simulink library "Lib_PF_LineEffAC_TMATS"  (R2017a)
settings: Solver=ode45  StartTime=0.0  StopTime=10.0  RelTol=1e-3  EnableMultiTasking=on
Description:
  | Thomas Modules
settings Model: Creator=jwchapm2  LastModifiedBy=glthoma1
settings DataIOCC: LimitDataPoints=on  SaveFormat=Array
settings OptimizationCC: ExpressionDepthLimit=2147483647  LifeSpan=inf
settings DebuggingCC: UnderspecifiedInitializationDetection=Classic  MergeDetectMultiDrivingBlocksExec=none  SolverPrmCheckMsg=warning  StateNameClashWarn=warning  SFUnexpectedBacktrackingDiag=warning  SFNoUnconditionalDefaultTransitionDiag=warning  SFExecutionAtInitializationDiag=none
settings HardwareCC: ProdBitPerPointer=32  ProdBitPerSizeT=32  ProdBitPerPtrDiffT=32  ProdLargestAtomicFloat=None  ProdIntDivRoundTo=Undefined  ProdEndianess=Unspecified  ProdWordSize=32  ProdHWDeviceType=32-bit Generic
settings ModelReferenceCC: PropagateSignalLabelsOutOfModel=off
settings GRTTargetCC: TargetLangStandard=C89/C90 (ANSI)  GeneratePreprocessorConditionals=Disable all
settings ConfigComp: CovMetricSettings=dw  CovHtmlReporting=on  CovSaveCumulativeToWorkspaceVar=on  CovSaveSingleToWorkspaceVar=on  CovExternalEMLEnable=off

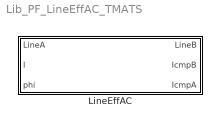
== system Lib_PF_LineEffAC_TMATS ==
  LineEffAC : Subsystem  mask{Eff_M=99}
      mask prompts: Eff_M "Eff_M - Efficiency, persent"
      mask Display:
      | fprintf('Efficiency\n %g %%',Eff_M)
      | port_label('input',1,'NodeA')
      | port_label('input',2,'IB')
      | port_label('input',3,'phiB')
      | port_label('output',1,'NodeB')
      | port_label('output',2,'IcmpB')
      | port_label('output',3,'IcmpA')

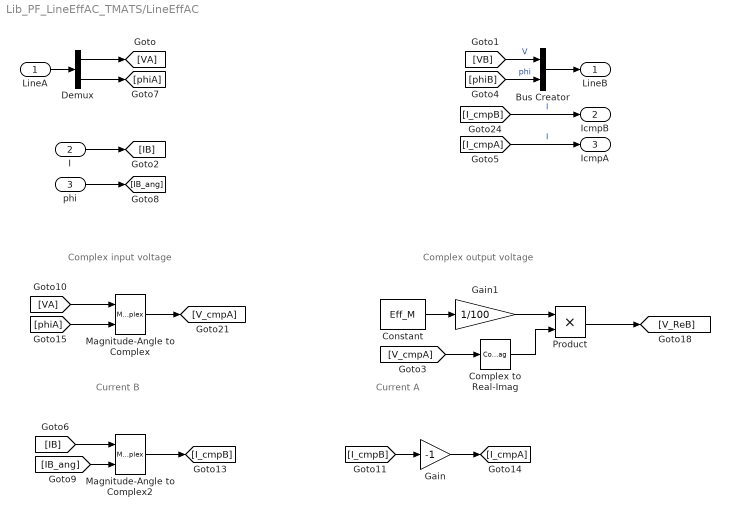
== system Lib_PF_LineEffAC_TMATS/LineEffAC ==
  note: Complex output voltage
  note: Complex input voltage
  note: Current B
  note: Current A
  LineA : Inport
  I : Inport  Port=2
  phi : Inport  Port=3
  Bus Creator : BusCreator  Inputs=2
  Complex to Real-Imag : ComplexToRealImag  Output=Real
  Constant : Constant  Value=Eff_M
  Demux : Demux  Outputs=2
  Gain : Gain  Gain=-1
  Gain1 : Gain  Gain=1/100
  Magnitude-Angle to Complex : MagnitudeAngleToComplex
  Magnitude-Angle to Complex2 : MagnitudeAngleToComplex
  Product : Product
  LineB : Outport
  IcmpB : Outport  Port=2
  IcmpA : Outport  Port=3
  wires:
  Demux/1 -> [VA]
  [phiB] -> Bus Creator/2  "phi"
  [I_cmpA] -> IcmpA/1  "I"
  phi/1 -> [IB_ang]
  Demux/2 -> [phiA]
  LineA/1 -> Demux/1
  I/1 -> [IB]
  [VB] -> Bus Creator/1  "V"
  Bus Creator/1 -> LineB/1
  [VA] -> Magnitude-Angle to Complex/1
  [phiA] -> Magnitude-Angle to Complex/2
  Magnitude-Angle to Complex/1 -> [V_cmpA]
  [I_cmpB] -> IcmpB/1  "I"
  [IB] -> Magnitude-Angle to Complex2/1
  [IB_ang] -> Magnitude-Angle to Complex2/2
  Magnitude-Angle to Complex2/1 -> [I_cmpB]
  [I_cmpB] -> Gain/1
  Gain/1 -> [I_cmpA]
  Constant/1 -> Gain1/1
  Gain1/1 -> Product/1
  [V_cmpA] -> Complex to Real-Imag/1
  Product/1 -> [V_ReB]
  Complex to Real-Imag/1 -> Product/2
